simulink model "tarea1_previous_version"  (R2022b)
settings: Solver=VariableStepAuto  StartTime=0.0  StopTime=0.3  RelTol=1e-3
libraries: spsMosfetLib x6, spsSeriesRLCBranchLib x6, eeTransforms x5, slpidlib x4, spsVoltageMeasurementLib x4, spsACVoltageSourceLib x3, spsCurrentMeasurementLib x3, spsPWMGenerator2LevelLib x2, spsDCVoltageSourceLib x1, spsGroundLib x1, spsPLL3phLib x1, spsPower3phInstantaneousLib x1
settings Model: Creator=PC  LastModifiedBy=Damian
settings OptimizationCC: ReuseModelBlockBuffer=on
settings RTWCC: GPUComputeCapability=5.0

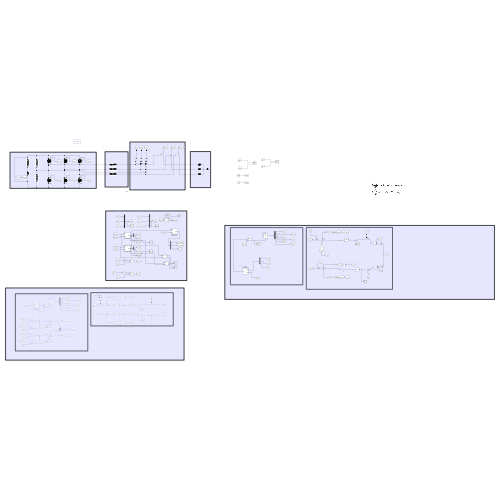
[thumbnail: Simulink's stored preview of the top-level diagram]
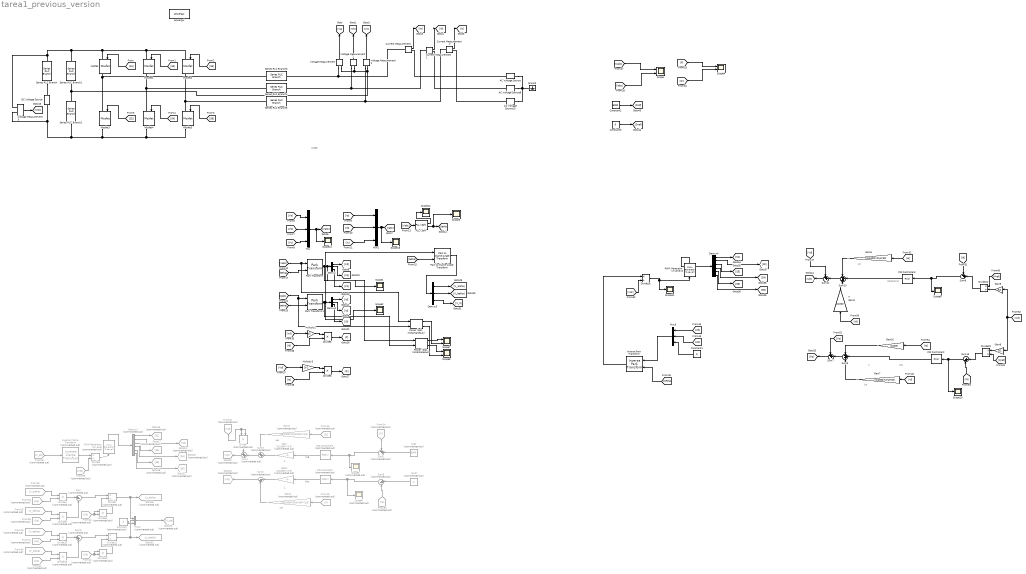
== system tarea1_previous_version ==
  note: 0.053
  note: L
  note: Viq
  note: Vid
  note: L
  note: Lw
  note: Lw
  note: Lw
  note: Viq
  note: R
  note: Control Id
  note: L
  note: Lw
  AC Voltage Source : spsACVoltageSourceLib/AC Voltage Source  Amplitude=240  Phase=0  Frequency=50  SampleTime=0  Measurements=None  BusType=swing  Pref=10e3  Qref=0  Qmin=-inf  Qmax=+inf
  AC Voltage Source10 : spsACVoltageSourceLib/AC Voltage Source  Amplitude=240  Phase=120  Frequency=50  SampleTime=0  Measurements=None  BusType=swing  Pref=10e3  Qref=0  Qmin=-inf  Qmax=+inf
  AC Voltage Source8 : spsACVoltageSourceLib/AC Voltage Source  Amplitude=240  Phase=-120  Frequency=50  SampleTime=0  Measurements=None  BusType=swing  Pref=10e3  Qref=0  Qmin=-inf  Qmax=+inf
  Constant : Constant  Commented=on  Value=0
  Constant1 : Constant  Value=0
  Constant2 : Constant  Value=5000
  Constant3 : Constant  Value=0
  Current Measurement : spsCurrentMeasurementLib/Current Measurement  PhasorSimulation=off  OutputType=Complex  PSBequivalent=0
  Current Measurement1 : spsCurrentMeasurementLib/Current Measurement  PhasorSimulation=off  OutputType=Complex  PSBequivalent=0
  Current Measurement2 : spsCurrentMeasurementLib/Current Measurement  PhasorSimulation=off  OutputType=Complex  PSBequivalent=0
  DC Voltage Source : spsDCVoltageSourceLib/DC Voltage Source  Amplitude=700  Measurements=None
  Demux : Demux  Outputs=3
  Demux1 : Demux  Outputs=3
  Demux2 : Demux  Commented=on  Outputs=6
  Demux3 : Demux  Outputs=3
  Demux4 : Demux  Outputs=6
  Divide{,1,8..10,12..13} (7 alike) : Product  Commented=on  Inputs=**
  Divide11 : Product  Commented=on  Inputs=*/
  Divide18 : Product  Inputs=*/
  Divide2 : Product  Commented=on  Inputs=*/
  Divide22 : Product  Inputs=*/
  Divide23 : Product  Inputs=/*
  Divide5 : Product  Inputs=**
  Divide6 : Product  Inputs=**
  Divide7 : Product  Commented=on  Inputs=*/
  From14 : From  Commented=on  GotoTag=P
  From16 : From  Commented=on  GotoTag=Q
  From18 : From  Commented=on  GotoTag=V_alpha
  From19 : From  Commented=on  GotoTag=P
  From22 : From  Commented=on  GotoTag=Vd
  From23 : From  Commented=on  GotoTag=Up
  From24 : From  Commented=on  GotoTag=Vd
  From25 : From  Commented=on  GotoTag=V_betha
  From26 : From  Commented=on  GotoTag=V_ab
  From29 : From  Commented=on  GotoTag=Vdc
  From30 : From  Commented=on  GotoTag=Q
  From39 : From  Commented=on  GotoTag=Uq
  From40 : From  Commented=on  GotoTag=V_betha
  From41 : From  Commented=on  GotoTag=Up
  From42 : From  Commented=on  GotoTag=Vd
  From43 : From  Commented=on  GotoTag=V_alpha
  From44 : From  Commented=on  GotoTag=Uq
  Gain : Gain  Commented=on  Gain=(2/1000)*(2/3)
  Gain1 : Gain  Commented=on  Gain=(2/1000)*(2/3)
  Gain10 : Gain  Gain=2/1000
  Gain2 : Gain  Commented=on  Gain=((2/1000)*2*pi*50)*(2/3)
  Gain3 : Gain  Gain=2/1000
  Gain4 : Gain  Commented=on  Gain=((2/1000)*2*pi*50)*(2/3)
  Gain6 : Gain  Gain=((2/1000)*2*pi*50)
  Gain7 : Gain  Gain=((2/1000)*2*pi*50)
  Gain8 : Gain  Gain=3/2
  Gain9 : Gain  Gain=3/2
  Goto12 : Goto  Commented=on  GotoTag=Up
  Goto13 : Goto  Commented=on  GotoTag=Uq
  Goto16 : Goto  Commented=on  GotoTag=S1
  Goto17 : Goto  Commented=on  GotoTag=S3
  Goto18 : Goto  Commented=on  GotoTag=S5
  Goto19 : Goto  Commented=on  GotoTag=S2
  Goto20 : Goto  Commented=on  GotoTag=S4
  Goto21 : Goto  Commented=on  GotoTag=S6
  Goto28 : Goto  Commented=on  GotoTag=u_alpha
  Goto32 : Goto  Commented=on  GotoTag=u_betha
  Goto33 : Goto  Commented=on  GotoTag=V_ab
  Ground : spsGroundLib/Ground  LConnTagsString=a
  Inverse Clarke Transform : eeTransforms/Inverse Clarke Transform  Commented=on  PowerInvariant=off
      settings: LibrarySourceBlock=|
      | ee_sl_lib/Mathematical
      | Transforms/Inverse
      | Clarke Transform
  Inverse Park Transform : eeTransforms/Inverse Park Transform  AxisAlignment=D-axis  PowerInvariant=off
      settings: LibrarySourceBlock=|
      | ee_sl_lib/Mathematical
      | Transforms/Inverse
      | Park Transform
  Mosfet{,1..5} (6 alike) : spsMosfetLib/Mosfet  Ron=0.1  Lon=0  Rd=0.01  Vfd=0  IC=0  Rs=1e5  Cs=inf  Measurements=on
  Multiply2 : Gain  Gain=3/2
  Multiply3 : Gain  Gain=3/-2
  Mux : Mux  Inputs=3
  Mux1 : Mux  Inputs=3
  Mux2 : Mux  Commented=on  Inputs=3
  Mux3 : Mux  Inputs=3
  PID Controller : slpidlib/PID Controller  Commented=on  Controller=PID  Form=Parallel  TimeDomain=Continuous-time  UseExternalTs=off  SampleTime=-1  IntegratorMethod=Forward Euler  FilterMethod=Forward Euler  ControllerParametersSource=internal  P=1  I=100  UseKiTs=off  D=0  N=100  UseFilter=on  TunerSelectOption=Transfer Function Based (PID Tuner App)  InitialConditionSource=internal  InitialConditionForIntegrator=0  InitialConditionForFilter=0  DifferentiatorICPrevScaledInput=0  ExternalReset=none  TrackingMode=off  Kt=1  LimitOutput=off  SatLimitsSource=internal  UpperSaturationLimit=inf  LowerSaturationLimit=-inf  LinearizeAsGain=on  AntiWindupMode=none  Kb=1  LimitIntegrator=off  UpperIntegratorSaturationLimit=inf  LowerIntegratorSaturationLimit=-inf  POutMin=[]  POutMax=[]  IOutMin=[]  IOutMax=[]  DOutMin=[]  DOutMax=[]  NOutMin=[]  NOutMax=[]  SumOutMin=[]  SumOutMax=[]  SaturationOutMin=[]  SaturationOutMax=[]  PParamMin=[]  PParamMax=[]  IParamMin=[]  IParamMax=[]  DParamMin=[]  DParamMax=[]  NParamMin=[]  NParamMax=[]  KbParamMin=[]  KbParamMax=[]  KtParamMin=[]  KtParamMax=[]  KbOutMin=[]  KbOutMax=[]  KtOutMin=[]  KtOutMax=[]  IntegratorOutMin=[]  IntegratorOutMax=[]  FilterOutMin=[]  FilterOutMax=[]  SumI1OutMin=[]  SumI1OutMax=[]  SumI2OutMin=[]  SumI2OutMax=[]  SumI3OutMin=[]  SumI3OutMax=[]  SumI4OutMin=[]  SumI4OutMax=[]  SumDOutMin=[]  SumDOutMax=[]  DifferentiatorOutMin=[]  DifferentiatorOutMax=[]  FilterDiffOutCoefMin=[]  FilterDiffOutCoefMax=[]  ReciprocalOutMin=[]  ReciprocalOutMax=[]  SumDenOutMin=[]  SumDenOutMax=[]  SumNumOutMin=[]  SumNumOutMax=[]  DivideOutMin=[]  DivideOutMax=[]  UdiffTsProdOutMin=[]  UdiffTsProdOutMax=[]  NTsProdOutMin=[]  NTsProdOutMax=[]  UintegralTsProdOutMin=[]  UintegralTsProdOutMax=[]  UngainTsProdOutMin=[]  UngainTsProdOutMax=[]  IntegratorContinuousStateAttributes=''  IntegratorStateMustResolveToSignalObject=off  IntegratorRTWStateStorageClass=Auto  FilterContinuousStateAttributes=''  FilterStateMustResolveToSignalObject=off  FilterRTWStateStorageClass=Auto  ParallelPVariant=InternalParameters  IdealPVariant=Disabled  IVariant=InternalParameters  DVariant=InternalParameters  IntegratorVariant=Continuous  SatVariant=Disabled  AWVariant=Passthrough  PCopyVariant=Disabled  TRVariant=Disabled  FdbkBlocksVariant=Forward  IdealPFdbkVariant=Disabled  SatFdbkVariant=Disabled  DerivativeFilterVariant=ContFilter  NVariant=InternalParameters  NCopyVariant=Disabled  FilterICVariant=InternalICsFilter  IntegratorICVariant=InternalICs  ExternalResetVariant=Disabled  TRSumVariant=Passthrough  SumFdbkVariant=Disabled  SumVariant=Sum_PID  TsampFilterVariant=InternalTs  TsampNgainVariant=Passthrough  TsampIntegralVariant=Disabled_SignalSpec  ExternalSaturationOutDataTypeStr=Inherit: Same as second input
  PID Controller1 : slpidlib/PID Controller  Commented=on  Controller=PID  Form=Parallel  TimeDomain=Continuous-time  UseExternalTs=off  SampleTime=-1  IntegratorMethod=Forward Euler  FilterMethod=Forward Euler  ControllerParametersSource=internal  P=1  I=100  UseKiTs=off  D=0  N=100  UseFilter=on  TunerSelectOption=Transfer Function Based (PID Tuner App)  InitialConditionSource=internal  InitialConditionForIntegrator=0  InitialConditionForFilter=0  DifferentiatorICPrevScaledInput=0  ExternalReset=none  TrackingMode=off  Kt=1  LimitOutput=off  SatLimitsSource=internal  UpperSaturationLimit=inf  LowerSaturationLimit=-inf  LinearizeAsGain=on  AntiWindupMode=none  Kb=1  LimitIntegrator=off  UpperIntegratorSaturationLimit=inf  LowerIntegratorSaturationLimit=-inf  POutMin=[]  POutMax=[]  IOutMin=[]  IOutMax=[]  DOutMin=[]  DOutMax=[]  NOutMin=[]  NOutMax=[]  SumOutMin=[]  SumOutMax=[]  SaturationOutMin=[]  SaturationOutMax=[]  PParamMin=[]  PParamMax=[]  IParamMin=[]  IParamMax=[]  DParamMin=[]  DParamMax=[]  NParamMin=[]  NParamMax=[]  KbParamMin=[]  KbParamMax=[]  KtParamMin=[]  KtParamMax=[]  KbOutMin=[]  KbOutMax=[]  KtOutMin=[]  KtOutMax=[]  IntegratorOutMin=[]  IntegratorOutMax=[]  FilterOutMin=[]  FilterOutMax=[]  SumI1OutMin=[]  SumI1OutMax=[]  SumI2OutMin=[]  SumI2OutMax=[]  SumI3OutMin=[]  SumI3OutMax=[]  SumI4OutMin=[]  SumI4OutMax=[]  SumDOutMin=[]  SumDOutMax=[]  DifferentiatorOutMin=[]  DifferentiatorOutMax=[]  FilterDiffOutCoefMin=[]  FilterDiffOutCoefMax=[]  ReciprocalOutMin=[]  ReciprocalOutMax=[]  SumDenOutMin=[]  SumDenOutMax=[]  SumNumOutMin=[]  SumNumOutMax=[]  DivideOutMin=[]  DivideOutMax=[]  UdiffTsProdOutMin=[]  UdiffTsProdOutMax=[]  NTsProdOutMin=[]  NTsProdOutMax=[]  UintegralTsProdOutMin=[]  UintegralTsProdOutMax=[]  UngainTsProdOutMin=[]  UngainTsProdOutMax=[]  IntegratorContinuousStateAttributes=''  IntegratorStateMustResolveToSignalObject=off  IntegratorRTWStateStorageClass=Auto  FilterContinuousStateAttributes=''  FilterStateMustResolveToSignalObject=off  FilterRTWStateStorageClass=Auto  ParallelPVariant=InternalParameters  IdealPVariant=Disabled  IVariant=InternalParameters  DVariant=InternalParameters  IntegratorVariant=Continuous  SatVariant=Disabled  AWVariant=Passthrough  PCopyVariant=Disabled  TRVariant=Disabled  FdbkBlocksVariant=Forward  IdealPFdbkVariant=Disabled  SatFdbkVariant=Disabled  DerivativeFilterVariant=ContFilter  NVariant=InternalParameters  NCopyVariant=Disabled  FilterICVariant=InternalICsFilter  IntegratorICVariant=InternalICs  ExternalResetVariant=Disabled  TRSumVariant=Passthrough  SumFdbkVariant=Disabled  SumVariant=Sum_PID  TsampFilterVariant=InternalTs  TsampNgainVariant=Passthrough  TsampIntegralVariant=Disabled_SignalSpec  ExternalSaturationOutDataTypeStr=Inherit: Same as second input
  PID Controller2 : slpidlib/PID Controller  Controller=PI  Form=Parallel  TimeDomain=Continuous-time  UseExternalTs=off  SampleTime=-1  IntegratorMethod=Forward Euler  FilterMethod=Forward Euler  ControllerParametersSource=internal  P=0.33  I=25  UseKiTs=off  D=0  N=100  UseFilter=on  TunerSelectOption=Transfer Function Based (PID Tuner App)  InitialConditionSource=internal  InitialConditionForIntegrator=0  InitialConditionForFilter=0  DifferentiatorICPrevScaledInput=0  ExternalReset=none  TrackingMode=off  Kt=1  LimitOutput=off  SatLimitsSource=internal  UpperSaturationLimit=0  LowerSaturationLimit=-400  LinearizeAsGain=on  AntiWindupMode=clamping  Kb=1  LimitIntegrator=off  UpperIntegratorSaturationLimit=inf  LowerIntegratorSaturationLimit=-inf  POutMin=[]  POutMax=[]  IOutMin=[]  IOutMax=[]  DOutMin=[]  DOutMax=[]  NOutMin=[]  NOutMax=[]  SumOutMin=[]  SumOutMax=[]  SaturationOutMin=[]  SaturationOutMax=[]  PParamMin=[]  PParamMax=[]  IParamMin=[]  IParamMax=[]  DParamMin=[]  DParamMax=[]  NParamMin=[]  NParamMax=[]  KbParamMin=[]  KbParamMax=[]  KtParamMin=[]  KtParamMax=[]  KbOutMin=[]  KbOutMax=[]  KtOutMin=[]  KtOutMax=[]  IntegratorOutMin=[]  IntegratorOutMax=[]  FilterOutMin=[]  FilterOutMax=[]  SumI1OutMin=[]  SumI1OutMax=[]  SumI2OutMin=[]  SumI2OutMax=[]  SumI3OutMin=[]  SumI3OutMax=[]  SumI4OutMin=[]  SumI4OutMax=[]  SumDOutMin=[]  SumDOutMax=[]  DifferentiatorOutMin=[]  DifferentiatorOutMax=[]  FilterDiffOutCoefMin=[]  FilterDiffOutCoefMax=[]  ReciprocalOutMin=[]  ReciprocalOutMax=[]  SumDenOutMin=[]  SumDenOutMax=[]  SumNumOutMin=[]  SumNumOutMax=[]  DivideOutMin=[]  DivideOutMax=[]  UdiffTsProdOutMin=[]  UdiffTsProdOutMax=[]  NTsProdOutMin=[]  NTsProdOutMax=[]  UintegralTsProdOutMin=[]  UintegralTsProdOutMax=[]  UngainTsProdOutMin=[]  UngainTsProdOutMax=[]  IntegratorContinuousStateAttributes=''  IntegratorStateMustResolveToSignalObject=off  IntegratorRTWStateStorageClass=Auto  FilterContinuousStateAttributes=''  FilterStateMustResolveToSignalObject=off  FilterRTWStateStorageClass=Auto  ParallelPVariant=InternalParameters  IdealPVariant=Disabled  IVariant=InternalParameters  DVariant=Disabled  IntegratorVariant=Continuous  SatVariant=Disabled  AWVariant=Passthrough  PCopyVariant=Disabled  TRVariant=Disabled  FdbkBlocksVariant=Forward  IdealPFdbkVariant=Disabled  SatFdbkVariant=Disabled  DerivativeFilterVariant=Disabled  NVariant=Disabled  NCopyVariant=Disabled_SignalSpec  FilterICVariant=Disabled  IntegratorICVariant=InternalICs  ExternalResetVariant=Disabled  TRSumVariant=Passthrough  SumFdbkVariant=Disabled  SumVariant=Sum_PI  TsampFilterVariant=InternalTs  TsampNgainVariant=Passthrough  TsampIntegralVariant=Disabled_SignalSpec  ExternalSaturationOutDataTypeStr=Inherit: Same as second input
  PID Controller3 : slpidlib/PID Controller  Controller=PI  Form=Parallel  TimeDomain=Continuous-time  UseExternalTs=off  SampleTime=-1  IntegratorMethod=Forward Euler  FilterMethod=Forward Euler  ControllerParametersSource=internal  P=0.33  I=50  UseKiTs=off  D=0  N=100  UseFilter=on  TunerSelectOption=Transfer Function Based (PID Tuner App)  InitialConditionSource=internal  InitialConditionForIntegrator=0  InitialConditionForFilter=0  DifferentiatorICPrevScaledInput=0  ExternalReset=none  TrackingMode=off  Kt=1  LimitOutput=off  SatLimitsSource=internal  UpperSaturationLimit=200  LowerSaturationLimit=0  LinearizeAsGain=on  AntiWindupMode=clamping  Kb=1  LimitIntegrator=off  UpperIntegratorSaturationLimit=inf  LowerIntegratorSaturationLimit=-inf  POutMin=[]  POutMax=[]  IOutMin=[]  IOutMax=[]  DOutMin=[]  DOutMax=[]  NOutMin=[]  NOutMax=[]  SumOutMin=[]  SumOutMax=[]  SaturationOutMin=[]  SaturationOutMax=[]  PParamMin=[]  PParamMax=[]  IParamMin=[]  IParamMax=[]  DParamMin=[]  DParamMax=[]  NParamMin=[]  NParamMax=[]  KbParamMin=[]  KbParamMax=[]  KtParamMin=[]  KtParamMax=[]  KbOutMin=[]  KbOutMax=[]  KtOutMin=[]  KtOutMax=[]  IntegratorOutMin=[]  IntegratorOutMax=[]  FilterOutMin=[]  FilterOutMax=[]  SumI1OutMin=[]  SumI1OutMax=[]  SumI2OutMin=[]  SumI2OutMax=[]  SumI3OutMin=[]  SumI3OutMax=[]  SumI4OutMin=[]  SumI4OutMax=[]  SumDOutMin=[]  SumDOutMax=[]  DifferentiatorOutMin=[]  DifferentiatorOutMax=[]  FilterDiffOutCoefMin=[]  FilterDiffOutCoefMax=[]  ReciprocalOutMin=[]  ReciprocalOutMax=[]  SumDenOutMin=[]  SumDenOutMax=[]  SumNumOutMin=[]  SumNumOutMax=[]  DivideOutMin=[]  DivideOutMax=[]  UdiffTsProdOutMin=[]  UdiffTsProdOutMax=[]  NTsProdOutMin=[]  NTsProdOutMax=[]  UintegralTsProdOutMin=[]  UintegralTsProdOutMax=[]  UngainTsProdOutMin=[]  UngainTsProdOutMax=[]  IntegratorContinuousStateAttributes=''  IntegratorStateMustResolveToSignalObject=off  IntegratorRTWStateStorageClass=Auto  FilterContinuousStateAttributes=''  FilterStateMustResolveToSignalObject=off  FilterRTWStateStorageClass=Auto  ParallelPVariant=InternalParameters  IdealPVariant=Disabled  IVariant=InternalParameters  DVariant=Disabled  IntegratorVariant=Continuous  SatVariant=Disabled  AWVariant=Passthrough  PCopyVariant=Disabled  TRVariant=Disabled  FdbkBlocksVariant=Forward  IdealPFdbkVariant=Disabled  SatFdbkVariant=Disabled  DerivativeFilterVariant=Disabled  NVariant=Disabled  NCopyVariant=Disabled_SignalSpec  FilterICVariant=Disabled  IntegratorICVariant=InternalICs  ExternalResetVariant=Disabled  TRSumVariant=Passthrough  SumFdbkVariant=Disabled  SumVariant=Sum_PI  TsampFilterVariant=InternalTs  TsampNgainVariant=Passthrough  TsampIntegralVariant=Disabled_SignalSpec  ExternalSaturationOutDataTypeStr=Inherit: Same as second input
  PLL (3ph) : spsPLL3phLib/PLL (3ph)  Fmin=45  Par_Init=[0, 50]  ParK=[180, 5000, 1]  TcD=1e-4  MaxRateChangeFreq=12  FilterCutOffFreq=25  Ts=0  AGC=on
  PWM Generator (2-Level) : spsPWMGenerator2LevelLib/PWM Generator (2-Level)  Commented=on  ModulatorType=Three-phase bridge (6 pulses)  ModulatorMode=Unsynchronized  Fc=27*60  Pc=90  nF=27  MinMax="[ -1  1 ]"  SamplingTechnique=Natural  ModulatingSignals=off  m=0.8  Freq=60  Phase=0  Ts=0  ShowCarrierOutport=off
  PWM Generator (2-Level)2 : spsPWMGenerator2LevelLib/PWM Generator (2-Level)  ModulatorType=Three-phase bridge (6 pulses)  ModulatorMode=Unsynchronized  Fc=27*60  Pc=90  nF=27  MinMax="[ -1  1 ]"  SamplingTechnique=Natural  ModulatingSignals=off  m=0.8  Freq=60  Phase=0  Ts=0  ShowCarrierOutport=off
  Park Transform : eeTransforms/Park Transform  AxisAlignment=Q-axis  PowerInvariant=off
      settings: LibrarySourceBlock=|
      | ee_sl_lib/Mathematical
      | Transforms/Park Transform
  Park Transform1 : eeTransforms/Park Transform  AxisAlignment=Q-axis  PowerInvariant=off
      settings: LibrarySourceBlock=|
      | ee_sl_lib/Mathematical
      | Transforms/Park Transform
  Park to Clarke Angle Transform : eeTransforms/Park to Clarke Angle Transform  AxisAlignment=Q-axis
      settings: LibrarySourceBlock=|
      | ee_sl_lib/Mathematical
      | Transforms/Park to Clarke
      | Angle Transform
  "Power (3ph, Instantaneous)" : spsPower3phInstantaneousLib/Power (3ph, Instantaneous)
  "Power (dq0, Instantaneous)" : spsPowerdq0InstantaneousLib/Power (dq0, Instantaneous)
      settings: LibrarySourceBlock=|
      | sps_lib/Sensors and Measurements/Power
      | (dq0, Instantaneous)
  Pref : Constant  Commented=on  Value=5000
  Qref : Constant  Commented=on  Value=0
  Scope{,4,7..8} (4 alike) : Scope  NumInputPorts=2
  Scope{1..3,9..14} (9 alike) : Scope
  Scope5 : Scope  Commented=on
  Scope6 : Scope  Commented=on
  Series RLC Branch : spsSeriesRLCBranchLib/Series RLC Branch  LConnTagsString=__new0  RConnTagsString=__new0  BranchType=R  Resistance=0.1  Inductance=0  SetiL0=off  InitialCurrent=0  Capacitance=0  Setx0=off  InitialVoltage=0  Measurements=None
  Series RLC Branch1 : spsSeriesRLCBranchLib/Series RLC Branch  LConnTagsString=__new0  RConnTagsString=__new0  BranchType=C  Resistance=0.1  Inductance=0  SetiL0=off  InitialCurrent=0  Capacitance=3000e-6  Setx0=off  InitialVoltage=0  Measurements=None
  Series RLC Branch2 : spsSeriesRLCBranchLib/Series RLC Branch  LConnTagsString=__new0  RConnTagsString=__new0  BranchType=C  Resistance=0.1  Inductance=0  SetiL0=off  InitialCurrent=0  Capacitance=3000e-6  Setx0=off  InitialVoltage=0  Measurements=None
  Series RLC Branch3 : spsSeriesRLCBranchLib/Series RLC Branch  LConnTagsString=__new0  RConnTagsString=__new0  BranchType=RL  Resistance=0.053  Inductance=2e-3  SetiL0=off  InitialCurrent=0  Capacitance=0  Setx0=off  InitialVoltage=0  Measurements=None
  Series RLC Branch4 : spsSeriesRLCBranchLib/Series RLC Branch  LConnTagsString=__new0  RConnTagsString=__new0  BranchType=RL  Resistance=0.053  Inductance=2e-3  SetiL0=off  InitialCurrent=0  Capacitance=0  Setx0=off  InitialVoltage=0  Measurements=None
  Series RLC Branch5 : spsSeriesRLCBranchLib/Series RLC Branch  LConnTagsString=__new0  RConnTagsString=__new0  BranchType=RL  Resistance=0.053  Inductance=2e-3  SetiL0=off  InitialCurrent=0  Capacitance=0  Setx0=off  InitialVoltage=0  Measurements=None
  Sum : Sum  Commented=on  Inputs=|+-
  Sum1 : Sum  Commented=on  Inputs=-+|
  Sum10 : Sum  Inputs=-++
  Sum11 : Sum  Inputs=++|
  Sum13 : Sum  Inputs=|+-
  Sum2 : Sum  Commented=on  Inputs=|-+
  Sum3 : Sum  Commented=on  Inputs=++|
  Sum4 : Sum  Commented=on  Inputs=++|
  Sum5 : Sum  Commented=on  Inputs=|++
  Sum6 : Sum  Commented=on  Inputs=|+-
  Sum7 : Sum  Inputs=++|
  Sum8 : Sum  Inputs=-+|
  Sum9 : Sum  Inputs=+++
  Voltage Measurement{,1..3} (4 alike) : spsVoltageMeasurementLib/Voltage Measurement  PhasorSimulation=off  OutputType=Complex  PSBequivalent=0
  powergui : spspowerguiLib/powergui  Priority=1  SimulationMode=Continuous  SampleTime=50e-6  frequency=60  Iterations=50  frequencyindice=50  Pbase=100e6  ErrMax=1e-4  UnitsV=kV  UnitsW=MW  buscounter=0  FunctionMessages=off  echomessages=off  EnableUseOfTLC=off  CurrentSourceSwitches=off  DisableSnubberDevices=off  DisableRonSwitches=off  DisableVfSwitches=off  DisplayEquations=off  AutomaticDiscreteSolvers=off  SolverType=Tustin/Backward Euler (TBE)  Interpol=off  ExternalGateDelay=off  methode=off  Ts=100  x0status=blocks  SPID=on  SwTol=0  HookPort=off  NonlinearTolerance=1e-4  nMaxIteration=100  ContinueOnMaxIteration=off  RestoreLinks=warning  ResistiveCurrentMeasurement=off  Frange=[0:2:500]  Ylog=off  Xlog=on  ShowGrid=off  save=off  variable=ZData  structure=0  ZoomFFT=off  StartTime=0.0  cycles=1  DisplayStyle=1  fundamental=60  FreqAxis=off  MaxFrequency=1000  frequencyindicesteady=1  RmsSteady=1  display=off
  wires:
  [S1] -> Mosfet/1
  [S3] -> Mosfet1/1
  [S5] -> Mosfet2/1
  [S6] -> Mosfet5/1
  [S4] -> Mosfet4/1
  [S2] -> Mosfet3/1
  Voltage Measurement/1 -> [Va]
  Voltage Measurement1/1 -> [Vb]
  Voltage Measurement2/1 -> [Vc]
  Current Measurement/1 -> [Ia]
  Current Measurement2/1 -> [Ic]
  Current Measurement1/1 -> [Ib]
  [Vc] -> Mux/3
  [Vb] -> Mux/2
  [Va] -> Mux/1
  [Ib] -> Mux1/2
  [Ic] -> Mux1/3
  [Ia] -> Mux1/1
  Mux/1 -> Scope12/1, [Vabc]
  Mux1/1 -> Scope13/1, [Iabc]
  [Vabc] -> "Power (3ph, Instantaneous)"/1, Park Transform/1
  Park Transform/1 -> "Power (dq0, Instantaneous)"/1, Scope1/1, Demux/1
  Pref/1 -> Sum1/2
  Demux/1 -> [Vd]
  Demux/2 -> [Vq]
  Demux1/2 -> [Iq]
  Park Transform1/1 -> "Power (dq0, Instantaneous)"/2, Park to Clarke Angle Transform/1, Scope2/1, Demux1/1
  Demux1/1 -> [Id]
  PID Controller/1 -> Gain1/1
  PID Controller1/1 -> Gain/1
  Gain2/1 -> Sum3/1
  From16/1 -> Gain2/1
  Gain/1 -> Sum3/2
  Gain1/1 -> Sum2/1
  From19/1 -> Gain4/1
  Gain4/1 -> Sum2/2
  Sum2/1 -> Goto13/1
  [Vabc] -> PLL (3ph)/1
  PLL (3ph)/2 -> Scope3/1, [tetha]
  [tetha] -> Park Transform/2
  [tetha] -> Park Transform1/2
  [Iabc] -> "Power (3ph, Instantaneous)"/2, Park Transform1/1
  Sum3/1 -> Sum4/2
  Sum4/1 -> Goto12/1
  Voltage Measurement3/1 -> [Vdc]
  PWM Generator (2-Level)/1 -> Demux2/1
  [Vabc] -> Scope/1
  [Iabc] -> Scope/2
  Demux1/3 -> [I0]
  Demux/3 -> [V0]
  Demux2/1 -> Goto16/1
  Demux2/2 -> Goto19/1
  Demux2/3 -> Goto17/1
  Demux2/4 -> Goto20/1
  Demux2/5 -> Goto18/1
  Demux2/6 -> Goto21/1
  [P] -> Scope4/1
  [Q] -> Scope4/2
  [Vd] -> Multiply3/1
  Divide5/1 -> [P]
  Divide6/1 -> [Q]
  Multiply3/1 -> Divide6/1
  Multiply2/1 -> Divide5/1
  [Id] -> Divide5/2
  [Iq] -> Divide6/2
  [Vd] -> Multiply2/1
  From14/1 -> Sum1/1
  Sum1/1 -> Scope5/1, PID Controller1/1
  Divide/1 -> Sum4/1
  From22/1 -> Divide/1, Divide/2
  [tetha] -> Park to Clarke Angle Transform/2
  Park to Clarke Angle Transform/1 -> Demux3/1
  Demux3/1 -> [V_alpha]
  Demux3/2 -> [V_betha]
  Demux3/3 -> [V_0]
  From18/1 -> Divide1/1
  From23/1 -> Divide1/2
  From24/1 -> Divide8/1, Divide8/2
  Divide8/1 -> Divide7/2
  From39/1 -> Divide9/2
  From25/1 -> Divide9/1
  Divide1/1 -> Sum/1
  Divide9/1 -> Sum/2
  Sum/1 -> Divide7/1
  Divide7/1 -> Mux2/1, Goto28/1
  Sum5/1 -> Divide11/1
  Divide10/1 -> Sum5/1
  Divide11/1 -> Goto32/1, Mux2/2
  From43/1 -> Divide13/1
  From42/1 -> Divide12/1, Divide12/2
  Divide13/1 -> Sum5/2
  From41/1 -> Divide10/2
  Divide12/1 -> Divide11/2
  From40/1 -> Divide10/1
  From44/1 -> Divide13/2
  Mux2/1 -> Goto33/1
  Constant/1 -> Mux2/3
  From26/1 -> Inverse Clarke Transform/1
  Inverse Clarke Transform/1 -> Divide2/1
  Divide2/1 -> PWM Generator (2-Level)/1
  Qref/1 -> Sum6/1
  From30/1 -> Sum6/2
  Sum6/1 -> Scope6/1, PID Controller/1
  From29/1 -> Divide2/2
  "Power (dq0, Instantaneous)"/1 -> Scope7/1
  "Power (dq0, Instantaneous)"/2 -> Scope8/1
  "Power (3ph, Instantaneous)"/1 -> Scope7/2
  "Power (3ph, Instantaneous)"/2 -> Scope8/2
  Constant2/1 -> [Pref]
  Constant3/1 -> [Qref]
  Sum11/1 -> [Ud]
  [tetha] -> Inverse Park Transform/2
  PWM Generator (2-Level)2/1 -> Demux4/1
  Demux4/1 -> [S1]
  Constant1/1 -> Mux3/3
  [Iq] -> Gain6/1
  Demux4/5 -> [S5]
  Mux3/1 -> Inverse Park Transform/1
  Gain9/1 -> Divide23/1
  [Qref] -> Divide23/2
  [Ud] -> Mux3/1
  Divide23/1 -> Sum13/1
  Divide22/1 -> Sum8/2
  [Id] -> Gain7/1
  Gain6/1 -> Sum10/1
  [Uq] -> Mux3/2
  Sum8/1 -> Scope9/1, PID Controller3/1
  Gain8/1 -> Divide22/2
  [Vd] -> Sum11/1
  [Pref] -> Divide22/1
  Inverse Park Transform/1 -> Divide18/1
  Demux4/3 -> [S3]
  PID Controller3/1 -> Sum10/2
  Sum10/1 -> Sum11/2
  Divide18/1 -> PWM Generator (2-Level)2/1, Scope11/1
  [Id] -> Sum8/1
  [Iq] -> Sum13/2
  Demux4/2 -> [S2]
  [Vdc] -> Divide18/2
  Sum13/1 -> PID Controller2/1, Scope10/1
  Demux4/4 -> [S4]
  [Vd] -> Gain9/1, Gain8/1
  Demux4/6 -> [S6]
  PLL (3ph)/1 -> Scope14/1
  Gain3/1 -> Sum10/3
  [Id] -> Gain3/1
  [Vq] -> Sum7/1
  Sum7/1 -> [Uq]
  Sum9/1 -> Sum7/2
  Gain7/1 -> Sum9/3
  Gain10/1 -> Sum9/1
  [Iq] -> Gain10/1
  PID Controller2/1 -> Sum9/2
  connections:
  Mosfet/RConn1 -- Mosfet3/LConn1 -- Series RLC Branch3/LConn1
  Mosfet1/RConn1 -- Mosfet4/LConn1 -- Series RLC Branch4/LConn1
  Mosfet2/RConn1 -- Series RLC Branch5/LConn1 -- Mosfet5/LConn1
  Series RLC Branch/LConn1 -- DC Voltage Source/RConn1
  Series RLC Branch2/LConn1 -- Voltage Measurement/LConn2 -- Voltage Measurement1/LConn2 -- Voltage Measurement2/LConn2 -- Series RLC Branch1/RConn1
  Series RLC Branch2/RConn1 -- Mosfet3/RConn1 -- Mosfet4/RConn1 -- Mosfet5/RConn1 -- DC Voltage Source/LConn1 -- Voltage Measurement3/LConn2
  Series RLC Branch/RConn1 -- Series RLC Branch1/LConn1 -- Mosfet/LConn1 -- Mosfet1/LConn1 -- Mosfet2/LConn1 -- Voltage Measurement3/LConn1
  AC Voltage Source10/LConn1 -- AC Voltage Source8/LConn1 -- AC Voltage Source/LConn1 -- Ground/LConn1
  AC Voltage Source/RConn1 -- Current Measurement/RConn1
  AC Voltage Source10/RConn1 -- Current Measurement2/RConn1
  AC Voltage Source8/RConn1 -- Current Measurement1/RConn1
  Current Measurement2/LConn1 -- Series RLC Branch5/RConn1 -- Voltage Measurement2/LConn1
  Current Measurement1/LConn1 -- Series RLC Branch4/RConn1 -- Voltage Measurement1/LConn1
  Current Measurement/LConn1 -- Series RLC Branch3/RConn1 -- Voltage Measurement/LConn1
